simulink subsystem "State_Machine"  (R2024b)
settings: Solver=VariableStepAuto  StartTime=0.0  StopTime=10.0  RelTol=1e-3
settings Model: Creator=alexa  LastModifiedBy=alexa

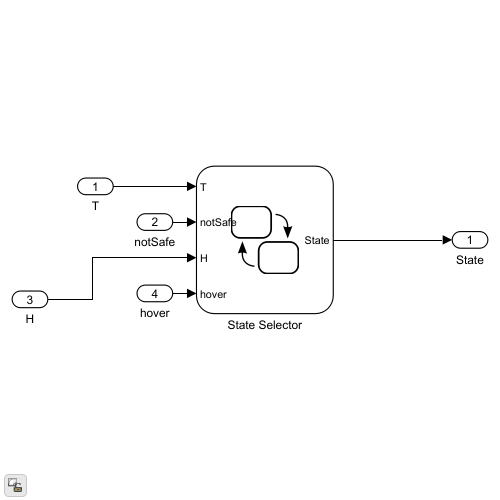
[thumbnail: Simulink's stored preview of the top-level diagram]
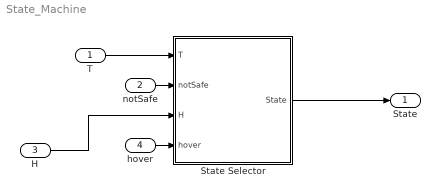
== system State_Machine ==
  T : Inport
  notSafe : Inport  Port=2
  H : Inport  Port=3
  hover : Inport  Port=4
  State Selector : Stateflow chart  TreatAsAtomicUnit=on
  State : Outport
  wires:
  State Selector/1(State) -> State/1
  T/1 -> State Selector/1(T)
  H/1 -> State Selector/3(H)
  notSafe/1 -> State Selector/2(notSafe)
  hover/1 -> State Selector/4(hover)

== stateflow chart State_Machine/State Selector ==
  state Landed
  state FollowPlan
  state EmergencyLanding
  state Hover
  (default) -> Landed
  Landed -> FollowPlan : [T > W || H > 0]
  Hover -> FollowPlan [order 1] : [hover == 0]
  FollowPlan -> Hover [order 2] : [hover == 1]
  FollowPlan -> EmergencyLanding [order 1] : [notSafe == 1]
  Hover -> EmergencyLanding [order 2] : [notSafe == 1]
  data: T input; W constant double =vehicle.m * g; notSafe input; State output Enum: StateEnum; H input; hover input
